simulink model "Q12"  (R2020b)
settings: Solver=VariableStepAuto  StartTime=0.0  StopTime=0.1  RelTol=1e-3
libraries: powerlib x16
settings Model: Creator=Huzai  LastModifiedBy=Huzai

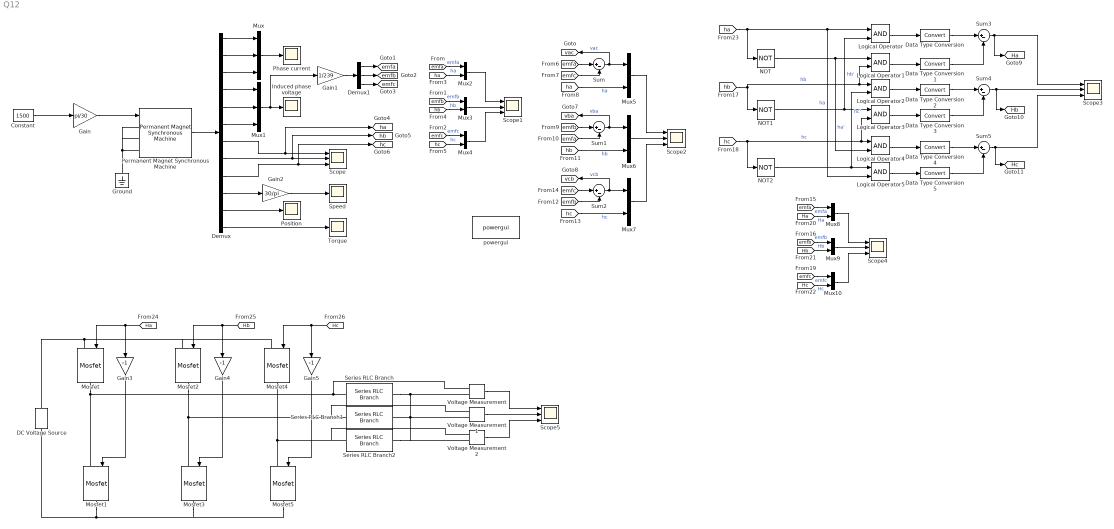
== system Q12 ==
  Constant : Constant  Value=1500
  DC Voltage Source : powerlib/Electrical Sources/DC Voltage Source  Amplitude=100  Measurements=None
  Data Type Conversion{,1..5} (6 alike) : DataTypeConversion
  Demux : Demux  Outputs=12
  Demux1 : Demux  Outputs=3
  Gain : Gain  Gain=pi/30
  Gain1 : Gain  Gain=1/239
  Gain2 : Gain  Gain=30/pi
  Gain3 : Gain  Gain=-1
  Gain4 : Gain  Gain=-1
  Gain5 : Gain  Gain=-1
  Ground : powerlib/Elements/Ground  LConnTagsString=a
  Induced phase voltage : Scope
  Logical Operator{,1..5} (6 alike) : Logic  AllPortsSameDT=off  OutDataTypeStr=boolean
  Mosfet{,1..5} (6 alike) : powerlib/Power Electronics/Mosfet  Ron=0.1  Lon=0  Rd=0.01  Vfd=0  IC=0  Rs=0.0001  Cs=inf  Measurements=off
  Mux : Mux  Inputs=3
  Mux1 : Mux  Inputs=3
  Mux{2..10} (9 alike) : Mux  Inputs=2
  NOT : Logic  Operator=NOT  IconShape=distinctive  AllPortsSameDT=off  OutDataTypeStr=boolean
  NOT1 : Logic  Operator=NOT  IconShape=distinctive  AllPortsSameDT=off  OutDataTypeStr=boolean
  NOT2 : Logic  Operator=NOT  IconShape=distinctive  AllPortsSameDT=off  OutDataTypeStr=boolean
  Permanent Magnet Synchronous Machine : powerlib/Machines/Permanent Magnet Synchronous Machine  NbPhases=3  FluxDistribution=Trapezoidal  RotorType=Round  MechanicalLoad=Speed w  PresetModel=No  ShowDetailedParameters=on  MeasurementBus=off  Resistance=8  Inductance=5.68e-3  dqInductances=[8.5e-3,8.5e-3]  La=0.000395  MachineConstant=Flux linkage established by magnets (V.s)  Flux=0.37973  VoltageCst=318.1219  TorqueCst=3.0378  Flat=120  Mechanical=[0.0027 0.0004924 4 0]  PolePairs=4  InitialConditions=[0,0, 0,0]  InitialConditions5ph=[0 0 0 0 0 0]  RefAngle=90 degrees behind phase A axis (modified Park)  IterativeDiscreteModel=Trapezoidal non iterative  TsBlock=-1  TsPowergui=0
  Phase current : Scope
  Position : Scope
  Scope{,1..5} (6 alike) : Scope  NumInputPorts=3
  Series RLC Branch : powerlib/Elements/Series RLC Branch  LConnTagsString=__new0  RConnTagsString=__new0  BranchType=R  Resistance=1000  Inductance=0  SetiL0=off  InitialCurrent=0  Capacitance=0  Setx0=off  InitialVoltage=0  Measurements=None
  Series RLC Branch1 : powerlib/Elements/Series RLC Branch  LConnTagsString=__new0  RConnTagsString=__new0  BranchType=R  Resistance=1000  Inductance=0  SetiL0=off  InitialCurrent=0  Capacitance=0  Setx0=off  InitialVoltage=0  Measurements=None
  Series RLC Branch2 : powerlib/Elements/Series RLC Branch  LConnTagsString=__new0  RConnTagsString=__new0  BranchType=R  Resistance=1000  Inductance=0  SetiL0=off  InitialCurrent=0  Capacitance=0  Setx0=off  InitialVoltage=0  Measurements=None
  Speed : Scope
  Sum{,1..5} (6 alike) : Sum  Inputs=|+-
  Torque : Scope
  Voltage Measurement : powerlib/Measurements/Voltage Measurement  PhasorSimulation=off  OutputType=Complex  PSBequivalent=0
  Voltage Measurement1 : powerlib/Measurements/Voltage Measurement  PhasorSimulation=off  OutputType=Complex  PSBequivalent=0
  Voltage Measurement2 : powerlib/Measurements/Voltage Measurement  PhasorSimulation=off  OutputType=Complex  PSBequivalent=0
  powergui : powerlib/powergui  Priority=1  SimulationMode=Continuous  SampleTime=50e-6  frequency=60  Iterations=50  frequencyindice=0  Pbase=100e6  ErrMax=1e-4  UnitsV=kV  UnitsW=MW  buscounter=0  FunctionMessages=off  echomessages=off  EnableUseOfTLC=off  CurrentSourceSwitches=off  DisableSnubberDevices=off  DisableRonSwitches=off  DisableVfSwitches=off  DisplayEquations=off  AutomaticDiscreteSolvers=off  SolverType=Tustin/Backward Euler (TBE)  Interpol=off  ExternalGateDelay=off  methode=off  Ts=100  x0status=blocks  SPID=on  SwTol=0  HookPort=off  NonlinearTolerance=1e-4  nMaxIteration=100  ContinueOnMaxIteration=off  RestoreLinks=warning  ResistiveCurrentMeasurement=off  Frange=[0:2:500]  Ylog=off  Xlog=on  ShowGrid=off  save=off  variable=ZData  structure=0  ZoomFFT=off  StartTime=0.0  cycles=1  DisplayStyle=1  fundamental=60  FreqAxis=off  MaxFrequency=1000  frequencyindicesteady=1  RmsSteady=1  display=off
  tag scope: Ha=global, Hb=global, Hc=global, emfa=global, emfb=global, emfc=global, ha=global, hb=global, hc=global, vac=global, vba=global, vcb=global
  wires:
  Gain/1 -> Permanent Magnet Synchronous Machine/1
  Constant/1 -> Gain/1
  Permanent Magnet Synchronous Machine/1 -> Demux/1
  Demux/1 -> Mux/1
  Demux/2 -> Mux/2
  Demux/3 -> Mux/3
  Demux/4 -> Mux1/1
  Demux/5 -> Mux1/2
  Demux/6 -> Mux1/3
  Mux/1 -> Phase current/1
  Mux1/1 -> Gain1/1, Induced phase voltage/1
  Gain1/1 -> Demux1/1
  Demux1/1 -> [emfa]
  Demux1/2 -> [emfb]
  Demux1/3 -> [emfc]
  Demux/8 -> [hb], Scope/2
  Demux/7 -> Scope/1, [ha]
  Demux/9 -> [hc], Scope/3
  Demux/10 -> Gain2/1
  Gain2/1 -> Speed/1
  Demux/11 -> Position/1
  Demux/12 -> Torque/1
  [emfa] -> Mux2/1  "emfa"
  [ha] -> Mux2/2  "ha"
  [emfb] -> Mux3/1  "emfb"
  [hb] -> Mux3/2  "hb"
  [emfc] -> Mux4/1  "emfc"
  [hc] -> Mux4/2  "hc"
  Mux2/1 -> Scope1/1
  Mux3/1 -> Scope1/2
  Mux4/1 -> Scope1/3
  [emfa] -> Sum/1
  [emfc] -> Sum/2
  Sum/1 -> [vac], Mux5/1  "vac"
  [ha] -> Mux5/2  "ha"
  Sum1/1 -> [vba], Mux6/1  "vba"
  [emfb] -> Sum1/1
  [emfa] -> Sum1/2
  [hb] -> Mux6/2  "hb"
  [emfb] -> Sum2/2
  [emfc] -> Sum2/1
  [hc] -> Mux7/2  "hc"
  Sum2/1 -> [vcb], Mux7/1  "vcb"
  Mux5/1 -> Scope2/1
  Mux7/1 -> Scope2/3
  Mux6/1 -> Scope2/2
  [hc] -> Logical Operator4/1, Logical Operator3/2, NOT2/1  "hc"
  NOT/1 -> Logical Operator4/2, Logical Operator1/1  "ha'"
  NOT1/1 -> Logical Operator3/1, Logical Operator/2  "hb'"
  NOT2/1 -> Logical Operator5/1, Logical Operator2/2  "hc'"
  [emfa] -> Mux8/1  "emfa"
  [ha] -> Logical Operator5/2, Logical Operator/1, NOT/1  "ha"
  [Hb] -> Mux9/2  "Hb"
  [Ha] -> Mux8/2  "Ha"
  [emfc] -> Mux10/1  "emfc"
  [emfb] -> Mux9/1  "emfb"
  [Hc] -> Mux10/2  "Hc"
  Mux8/1 -> Scope4/1
  [hb] -> Logical Operator1/2, Logical Operator2/1, NOT1/1  "hb"
  Mux10/1 -> Scope4/3
  Mux9/1 -> Scope4/2
  Sum5/1 -> Scope3/3, [Hc]
  Sum3/1 -> Scope3/1, [Ha]
  Sum4/1 -> [Hb], Scope3/2
  Logical Operator/1 -> Data Type Conversion/1
  Data Type Conversion/1 -> Sum3/1
  Logical Operator1/1 -> Data Type Conversion1/1
  Data Type Conversion1/1 -> Sum3/2
  Logical Operator2/1 -> Data Type Conversion2/1
  Data Type Conversion2/1 -> Sum4/1
  Logical Operator3/1 -> Data Type Conversion3/1
  Data Type Conversion3/1 -> Sum4/2
  Logical Operator4/1 -> Data Type Conversion4/1
  Data Type Conversion4/1 -> Sum5/1
  Logical Operator5/1 -> Data Type Conversion5/1
  Data Type Conversion5/1 -> Sum5/2
  [Ha] -> Gain3/1, Mosfet/1
  Gain3/1 -> Mosfet1/1
  Gain4/1 -> Mosfet3/1
  [Hb] -> Gain4/1, Mosfet2/1
  [Hc] -> Gain5/1, Mosfet4/1
  Gain5/1 -> Mosfet5/1
  Voltage Measurement1/1 -> Scope5/2
  Voltage Measurement/1 -> Scope5/1
  Voltage Measurement2/1 -> Scope5/3
  connections:
  Permanent Magnet Synchronous Machine/LConn3 -- Permanent Magnet Synchronous Machine/LConn1 -- Permanent Magnet Synchronous Machine/LConn2 -- Ground/LConn1
  Mosfet1/RConn1 -- Mosfet3/RConn1 -- Mosfet5/RConn1 -- DC Voltage Source/LConn1
  DC Voltage Source/RConn1 -- Mosfet4/LConn1 -- Mosfet2/LConn1 -- Mosfet/LConn1
  Mosfet/RConn1 -- Mosfet1/LConn1 -- Voltage Measurement/LConn1 -- Series RLC Branch/LConn1
  Mosfet2/RConn1 -- Mosfet3/LConn1 -- Voltage Measurement1/LConn1 -- Series RLC Branch1/LConn1
  Mosfet5/LConn1 -- Voltage Measurement2/LConn1 -- Series RLC Branch2/LConn1 -- Mosfet4/RConn1
  Series RLC Branch/RConn1 -- Voltage Measurement/LConn2 -- Voltage Measurement2/LConn2 -- Series RLC Branch2/RConn1 -- Voltage Measurement1/LConn2 -- Series RLC Branch1/RConn1
